simulink model "PV_generator_sim"  (R2019b)
settings: Solver=VariableStepAuto  StartTime=0.0  StopTime=120  RelTol=1e-3
values from neighbouring files (symbols this model uses):
  A = A1*duty+A2*(1-duty)    [statespaceLQRsetup.m]    (also in statespace_ackerman_setup.m)
  B = [1/L;0]    [statespaceLQRsetup.m]    (also in statespace_ackerman_setup.m)
  C_eq = 500e-6    (= 0.0005)    [statespaceLQRsetup.m]    (also in statespace_ackerman_setup.m)
  C_state = [1 0; ((1-duty)*(R*R_c)/(R+R_c)) R/(R+R_c)]    [statespaceLQRsetup.m]    (also in statespace_ackerman_setup.m)
  D = [0;0]    [statespaceLQRsetup.m]    (also in statespace_ackerman_setup.m)
  K = place(A,B,eigs)    [statespace_ackerman_setup.m]
  K_r = -1/([1 0 0]*inv(A-B*K)*B)    [statespaceLQRsetup.m]    (also in statespace_ackerman_setup.m = -1/([((1-duty)*(R*R_c)/(R+R_c)) R/(R+R_c)]*inv(A-B*K)*B))
undefined symbols (not defined in the file or in its folder): Ion, Lithium, Vnom_dc
libraries: powerlib x9, simulink x2, electricdrivelib x1, re_lib x1, eePwmGenerator x1
settings Model: SimulationMode=accelerator  Creator=SPS VISION  LastModifiedBy=SPS VISION
settings SolverCC: ZeroCrossAlgorithm=Adaptive
settings DebuggingCC: IgnoredZcDiagnostic=none

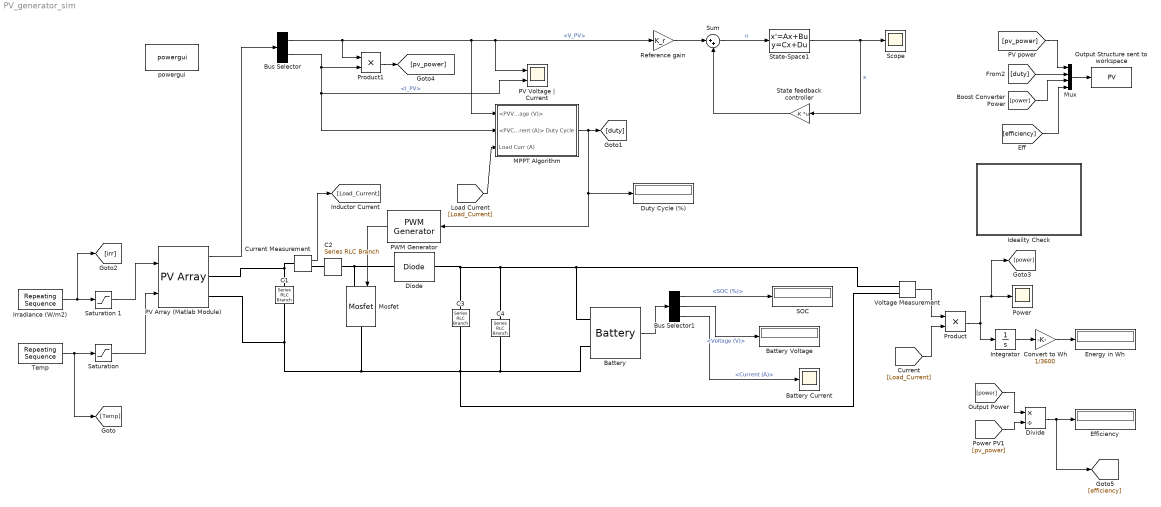
== system PV_generator_sim ==
  Battery : electricdrivelib/Extra Sources/Battery  BatType=Lithium-Ion  ShowTempParam=off  ThermalPreset=no  ShowAgeParam=off  NomV=48  NomQ=120  SOC=0  Batt_Tr=2  PresetModel=on  MaxQ=120  MinV=36  FullV=55.8714  Dis_rate=52.1739  R=0.004  Normal_OP=108.5217  expZone="[51.8585      5.89565]"  current=[6.5 13 32.5]  Units=Time  Tci=20  NomT=20  T2=-30  MaxQ2=4.8  FullV2=7.1  Normal_OP2=5.655  expZone2="[6.58           1]"  Rca=0.6  ti=2000  Dp=0  Neq0=0  Tsim=1e6  Ta1=25  Qeol=5.4*0.9  Reol=0.013333*1.2  Char_age=[2.3478, 3]  Dis_age=[2.3478, 10]  N1=1500  N2=10500  N3=1000  N4=1400  Ta2=45  N5=950
      settings: SourceProductName=Simscape Electrical
  Battery Current : Scope
  "Battery Voltage " : Display
  Bus Selector : BusSelector  OutputSignals=V_PV,I_PV
  Bus Selector1 : BusSelector  OutputSignals=SOC (%),Voltage (V),Current (A)
  C1 : powerlib/Elements/Series RLC Branch  LConnTagsString=__new0  RConnTagsString=__new0  BranchType=RC  Resistance=0.0001  Inductance=1.0  SetiL0=off  InitialCurrent=0  Capacitance=500e-6  Setx0=off  InitialVoltage=Vnom_dc/2  Measurements=None
      settings: SourceProductName=Simscape Electrical
  C2 : powerlib/Elements/Series RLC Branch  LConnTagsString=__new0  RConnTagsString=__new0  BranchType=RL  Resistance=0.1  Inductance=0.01  SetiL0=off  InitialCurrent=0  Capacitance=C_eq  Setx0=off  InitialVoltage=Vnom_dc/2  Measurements=Branch current
      settings: SourceProductName=Simscape Electrical
  C3 : powerlib/Elements/Series RLC Branch  LConnTagsString=__new0  RConnTagsString=__new0  BranchType=RC  Resistance=0.0001  Inductance=1.0  SetiL0=off  InitialCurrent=0  Capacitance=500e-6  Setx0=off  InitialVoltage=Vnom_dc/2  Measurements=Branch voltage
      settings: SourceProductName=Simscape Electrical
  C4 : powerlib/Elements/Series RLC Branch  LConnTagsString=__new0  RConnTagsString=__new0  BranchType=R  Resistance=20  Inductance=1.0  SetiL0=off  InitialCurrent=0  Capacitance=C_eq  Setx0=off  InitialVoltage=Vnom_dc/2  Measurements=Branch voltage and current
      settings: SourceProductName=Simscape Electrical
  Convert to Wh : Gain  Gain=1/3600
  Current Measurement : powerlib/Measurements/Current Measurement  PhasorSimulation=off  OutputType=Complex  PSBequivalent=0
      settings: SourceProductName=Simscape Electrical
  Diode : powerlib/Power Electronics/Diode  Ron=0.001  Lon=0  Vf=0.8  IC=0  UseSnubber=0  Rs=500  Cs=250e-9  Measurements=off
      settings: SourceProductName=Simscape Electrical
  Divide : Product  Inputs=*/
  Duty Cycle (%) : Display
  Efficiency : Display
  Energy in Wh : Display
  Ideality Check : Subsystem
  Integrator : Integrator
  "Irradiance (W/m2) " : simulink/Sources/Repeating Sequence  rep_seq_t=[0 10 20 30 40 50 60 70 80 90 100 110 120]  rep_seq_y=[100 400 550 700 700 800 800 750 600 500 400 200 200]
  MPPT Algorithm : Subsystem
  Mosfet : powerlib/Power Electronics/Mosfet  Ron=0.1  Lon=0  Rd=0.01  Vfd=0  IC=0  Rs=inf  Cs=0  Measurements=off
      settings: SourceProductName=Simscape Electrical
  Mux : Mux
  Output Structure sent to workspace : ToWorkspace  VariableName=PV  SaveFormat=Structure With Time  SampleTime=-1
  PV Array (Matlab Module) : re_lib/Solar/PV Array  Npar=2  Nser=2  PlotType=array @ 1000 W/m2 & specified temperatures  S_vec="[ 1000  500  100 ]"  Temp_C_vec=[20]  ModuleName=Silray API-230P(60)-XH  PlotWhenSelected=off  Pm=230.1168  Ncell=60  Voc=36.96  Isc=8.3  Vm=30.12  Im=7.64  beta_Voc_pc=-0.3664  alpha_Isc_pc=0.073699  beta_Voc=-0.13542  alpha_Isc=0.006117  IL=8.3202  I0=3.5447e-10  nI=1.0056  Rsh=120.6455  Rs=0.29304  BAL=on  Tc=1e-6  Tfilter=5e-5
      settings: SourceProductName=Simscape Electrical
  PV Voltage | Current : Scope  NumInputPorts=2
  PWM Generator : eePwmGenerator/PWM Generator  CarrCount=Up  Tper=0.001  Ts=5e-5
      settings: SourceProductName=Simscape Electrical
  Power : Scope
  Product : Product
  Product1 : Product
  Reference gain : Gain  Gain=K_r
  SOC : Display
  "Saturation " : Saturate  UpperLimit=55  LowerLimit=5
  Saturation 1 : Saturate  UpperLimit=1308  LowerLimit=0
  Scope : Scope
  State feedback controller : Gain  Gain=-K  Multiplication=Matrix(K*u)
  State-Space1 : StateSpace  A=A  B=B  C=C_state  D=D  InitialCondition=0
  Sum : Sum  Inputs=|++
  "Temp " : simulink/Sources/Repeating Sequence  rep_seq_t=[0 10 20 30 40 50 60 70 80 90 100 110 120]  rep_seq_y=[10 11 14 16 18 20 20 19 17 15 14 10 8]
  Voltage Measurement : powerlib/Measurements/Voltage Measurement  PhasorSimulation=off  OutputType=Complex  PSBequivalent=0
      settings: SourceProductName=Simscape Electrical
  powergui : powerlib/powergui  Priority=1  SimulationMode=Discrete  SampleTime=1e-05  frequency=60  Iterations=50  frequencyindice=0  Pbase=100e6  ErrMax=1e-4  UnitsV=kV  UnitsW=MW  buscounter=0  FunctionMessages=off  echomessages=off  EnableUseOfTLC=off  CurrentSourceSwitches=off  DisableSnubberDevices=off  DisableRonSwitches=off  DisableVfSwitches=off  DisplayEquations=off  AutomaticDiscreteSolvers=off  SolverType=Tustin/Backward Euler (TBE)  Interpol=off  ExternalGateDelay=off  methode=off  Ts=100  x0status=blocks  SPID=on  SwTol=0  HookPort=off  NonlinearTolerance=1e-4  nMaxIteration=100  ContinueOnMaxIteration=off  RestoreLinks=warning  ResistiveCurrentMeasurement=off  Frange=[0:2:500]  Ylog=off  Xlog=on  ShowGrid=off  save=off  variable=ZData  structure=0  ZoomFFT=off  StartTime=0.0  cycles=1  DisplayStyle=1  fundamental=60  FreqAxis=off  MaxFrequency=1000  frequencyindicesteady=1  RmsSteady=1  display=off
      settings: SourceProductName=Simscape Electrical
  wires:
  "Irradiance (W/m2) "/1 -> [irr], Saturation 1/1
  "Saturation "/1 -> PV Array (Matlab Module)/2
  Saturation 1/1 -> PV Array (Matlab Module)/1
  "Temp "/1 -> [Temp], "Saturation "/1
  PV Array (Matlab Module)/1 -> Bus Selector/1
  PWM Generator/1 -> Mosfet/1
  Mux/1 -> Output Structure sent to workspace/1
  State-Space1/1 -> State feedback controller/1, Scope/1  "x"
  State feedback controller/1 -> Sum/2
  Reference gain/1 -> Sum/1
  Sum/1 -> State-Space1/1  "u"
  Battery/1 -> Bus Selector1/1
  MPPT Algorithm/1(Duty Cycle) -> PWM Generator/1, Duty Cycle (%)/1, [duty]
  Bus Selector1/2 -> "Battery Voltage "/1  "<Voltage (V)>"
  Bus Selector1/1 -> SOC/1  "<SOC (%)>"
  Current Measurement/1 -> [Load_Current]
  Bus Selector1/3 -> Battery Current/1  "<Current (A)>"
  Voltage Measurement/1 -> Product/1
  [Load_Current] -> Product/2
  Product/1 -> Integrator/1, [power], Power/1
  Integrator/1 -> Convert to Wh/1
  Convert to Wh/1 -> Energy in Wh/1
  Product1/1 -> [pv_power]
  [pv_power] -> Divide/2
  [power] -> Divide/1
  Divide/1 -> [efficiency], Efficiency/1
  [efficiency] -> Mux/4
  [power] -> Mux/3
  [pv_power] -> Mux/1
  [duty] -> Mux/2
  [Load_Current] -> MPPT Algorithm/3(Load Curr (A))
  Bus Selector/1 -> MPPT Algorithm/1(<PVVoltage (V)>), PV Voltage | Current/1, Reference gain/1, Product1/1  "<V_PV>"
  Bus Selector/2 -> MPPT Algorithm/2(<PVCurrent (A)>), PV Voltage | Current/2, Product1/2  "<I_PV>"
  connections:
  PV Array (Matlab Module)/RConn2 -- C3/RConn1 -- Voltage Measurement/LConn2 -- C4/RConn1 -- Battery/LConn2 -- Mosfet/RConn1 -- C1/RConn1
  Diode/LConn1 -- Mosfet/LConn1 -- C2/RConn1
  PV Array (Matlab Module)/RConn1 -- Current Measurement/LConn1 -- C1/LConn1
  Diode/RConn1 -- C3/LConn1 -- C4/LConn1 -- Battery/LConn1 -- Voltage Measurement/LConn1
  Current Measurement/RConn1 -- C2/LConn1

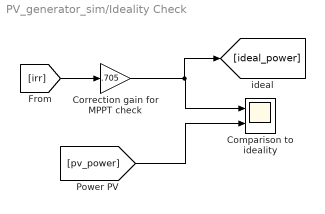
== system PV_generator_sim/Ideality Check ==
  Comparison to ideality : Scope  NumInputPorts=2
  Correction gain for MPPT check : Gain  Gain=.705
  wires:
  [pv_power] -> Comparison to ideality/2
  [irr] -> Correction gain for MPPT check/1
  Correction gain for MPPT check/1 -> [ideal_power], Comparison to ideality/1

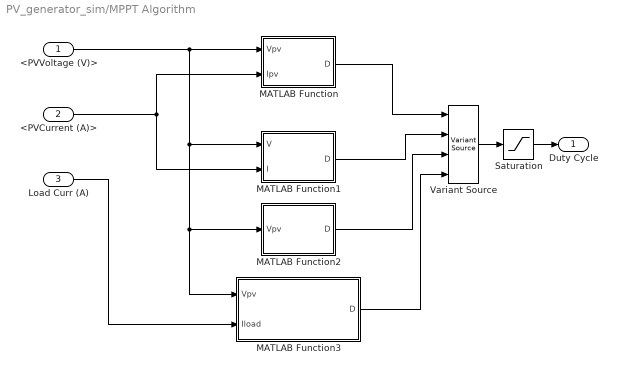
== system PV_generator_sim/MPPT Algorithm ==
  <PVVoltage (V)> : Inport
  <PVCurrent (A)> : Inport  Port=2
  Load Curr (A) : Inport  Port=3
  MATLAB Function : MATLAB Function  TreatAsAtomicUnit=on
  MATLAB Function1 : MATLAB Function  TreatAsAtomicUnit=on
  MATLAB Function2 : MATLAB Function  TreatAsAtomicUnit=on
  MATLAB Function3 : MATLAB Function  TreatAsAtomicUnit=on
  "Saturation " : Saturate  UpperLimit=1  LowerLimit=0
  Variant Source : VariantSource  VariantControlMode=Label  LabelModeActiveChoice=P&O
  Duty Cycle : Outport
  wires:
  <PVVoltage (V)>/1 -> MATLAB Function3/1(Vpv), MATLAB Function2/1(Vpv), MATLAB Function1/1(V), MATLAB Function/1(Vpv)
  <PVCurrent (A)>/1 -> MATLAB Function/2(Ipv), MATLAB Function1/2(I)
  MATLAB Function/1(D) -> Variant Source/1
  Variant Source/1 -> "Saturation "/1
  MATLAB Function1/1(D) -> Variant Source/2
  MATLAB Function2/1(D) -> Variant Source/3
  "Saturation "/1 -> Duty Cycle/1
  Load Curr (A)/1 -> MATLAB Function3/2(Iload)
  MATLAB Function3/1(D) -> Variant Source/4

== matlab function PV_generator_sim/MPPT Algorithm/MATLAB Function1 ==
  settings: updateMethod=DISCRETE
  data: V input; D output; I input
function D = IncCond(V,I)
Dinit = 0.05;  %Initial value for D output
Dmax = 1;   %Maximum value for D
Dmin = 0;   %Minimum value for D
deltaD = 0.005; %Increment value used to increase/decrease the duty cycle D

  
persistent Vold Pold Dold M Iold;

dataType = 'double';

if isempty(Vold)
    Vold=0;
    Pold=0;
    Iold=0;
    Dold=Dinit;
    M=1;
end
P= V*I;
dV= V - Vold;
dP= P - Pold;
dI= I - Iold;
M=abs(dP);

if M < 0.005
    D=Dold;
else
    if dV == 0
        if dI == 0
            D=Dold;
        elseif dI>0
            D=Dold - (M*deltaD);
        else 
            D=Dold + (M*deltaD);
        end    
    else
        if dI/dV == -I/V
            D=Dold;
        elseif dI/dV>-I/V    
           D=Dold - (M*deltaD);
        else
           D=Dold + (M*deltaD);  
        end  
    end    
end

if D >= Dmax | D<= Dmin
    D=Dold;
end

Dold=D;
Vold=V;
Pold=P;
Iold=I;

== matlab function PV_generator_sim/MPPT Algorithm/MATLAB Function ==
  settings: updateMethod=DISCRETE
  data: Vpv input; D output; Ipv input
function D = PandO(Vpv,Ipv)

% incremental duty cycle change
delta_D = 0.005;

% grabs workspace variables or initializes them below
persistent Dprev Pprev Vprev

if isempty(Dprev)
    Dprev = 0.01;
    Vprev = 0;
    Pprev = 0;
end

% Calculate measured array power
Ppv = Vpv*Ipv;

% Increase or decrease duty cycle based on conditions
if (Ppv-Pprev) ~= 0
    if (Ppv-Pprev) > 0
        if (Vpv-Vprev) > 0
            D = Dprev - delta_D;
        else
            D = Dprev + delta_D;
        end
    else
        if (Vpv-Vprev) > 0
            D = Dprev + delta_D;
        else
            D = Dprev - delta_D;
        end        
    end
else
    D = Dprev;
end
if D<0
    D=0;
end
if D>1
    D=1;
end
% Update internal values
Dprev = D;
Vprev = Vpv;
Pprev = Ppv;

== matlab function PV_generator_sim/MPPT Algorithm/MATLAB Function2 ==
  settings: updateMethod=DISCRETE
  data: Vpv input; D output
function D = ConstVolt(Vpv)

% incremental duty cycle change
delta_d = 0.005;

% grabs workspace variables or initializes them below
persistent Dprev Vprev

if isempty(Dprev)
    Dprev = 0.01;
    Vprev = 0;
end
Voc = 36.7;
Vref = 0.76*Voc;

% Increase or decrease duty cycle based on conditions
if abs(Vref - Vpv)<44
    D = Dprev;
else
    if Vpv>Vref
        D = Dprev+delta_d;
    else
        D = Dprev - delta_d;
    end
end

% Update internal values
Dprev = D;
Vprev = Vpv;

== matlab function PV_generator_sim/MPPT Algorithm/MATLAB Function3 ==
  settings: updateMethod=DISCRETE
  data: Vpv input; D output; Iload input
function D = CurrentSweep(Vpv,Iload)

% incremental duty cycle change
delta_d = 0.0005;
delta_t=1/100000;
% grabs workspace variables or initializes them below
persistent Dprev Vprev Iprev

if isempty(Dprev)
    Dprev = 0.01;
    Vprev = 0;
    Iprev = 0;
end

dVpv = (Vpv-Vprev)/delta_t;
dIload = (Iload - Iprev)/delta_t;

% Increase or decrease duty cycle based on conditions
% Increase or decrease duty cycle based on conditions
if abs(dVpv)<3300
    D = Dprev;
else
    if sign(dIload) && sign(dVpv)
        D=Dprev+delta_d; 
    else
        D=Dprev-delta_d; 
    end    
end
% Update internal values
Dprev = D;
Vprev = Vpv;
Iprev = Iload;
